simulink model "ROS2ValetPathPlannerExample"  (R2022b)
settings: Solver=FixedStepAuto  StartTime=0.0  StopTime=inf  RelTol=1e-3
model workspace (MAT data in the model file):
  SL_ROS_VariableLengthArrays_MaxSizes.CommonInfo.ArrayTruncateAction = 'EmitWarning'
  SL_ROS_VariableLengthArrays_MaxSizes.MsgTypeMap = containers.Map
  SL_ROS_VariableLengthArrays_MaxSizes.MsgTypeMap.serialization.keys = {'std_msgs/Float64MultiArray'}
  SL_ROS_VariableLengthArrays_MaxSizes.MsgTypeMap.serialization.values{1}.PropertyName = 'data'
  SL_ROS_VariableLengthArrays_MaxSizes.MsgTypeMap.serialization.values{1}.DataType = 'double'
  SL_ROS_VariableLengthArrays_MaxSizes.MsgTypeMap.serialization.values{1}.MaxLength = 1500
  SL_ROS_VariableLengthArrays_MaxSizes.MsgTypeMap.serialization.uniformity = 0
  SL_ROS_VariableLengthArrays_MaxSizes.MsgTypeMap.serialization.keyType = 'char'
  SL_ROS_VariableLengthArrays_MaxSizes.MsgTypeMap.serialization.valueType = 'any'
values from neighbouring files (symbols this model uses):
  costmap = vehicleCostmap(combinedMap, 'CellSize', res)    [exampleHelperROSValetSLCreateCostmap.m]    (also in exampleHelperROSValetSLVisualizePath.m = vehicleCostmap(costmapStruct.Costs,          'FreeThreshold')
  costmapStruct = rmfield(costmapStruct, 'CollisionChecker')    [exampleHelperROSValetSLCreateUtilityStruct.m]
  directions = obj.DirectionsInternal    [ExampleHelperROSValetPathAnalyzer.m]
  vehicleDimsStruct = exampleHelperROSValetMatchStructFields(vehicleDimsStruct, obj.CollisionChecker.VehicleDimensions)    [exampleHelperROSValetSLCreateUtilityStruct.m]
undefined symbols (not defined in the file or in its folder): data, data_SL_Info
libraries: ros2lib x13, drivinglib x2, helperVarsizeLib x1, simulink x1
settings Model: Creator=The MathWorks, Inc.  LastModifiedBy=The MathWorks, Inc.
settings SolverCC: AlgebraicLoopSolver=TrustRegion
settings OptimizationCC: EnhancedBackFolding=on  PassReuseOutputArgsAs=Individual arguments  ZeroExternalMemoryAtStartup=off  ZeroInternalMemoryAtStartup=off  MaxStackSize=64  OptimizeBlockOrder=speed  DifferentSizesBufferReuse=on  OptimizationCustomize=off  EfficientTunableParamExpr=on
settings DebuggingCC: ParameterTunabilityLossMsg=error  UnconnectedInputMsg=warning  UnconnectedOutputMsg=warning  UnconnectedLineMsg=warning  SFMachineParentedDataDiag=warning
settings ModelReferenceCC: EnableRefExpFcnMdlSchedulingChecks=on
settings SFSimCC: SimTargetLang=C++
settings RTWCC: Description=Embedded Coder  SystemTargetFile=ert.tlc  HardwareBoard=Robot Operating System 2 (ROS 2)  TLCOptions=-aInlineSetEventsForThisBaseRateFcn=TLC_FALSE -aSuppressMultiTaskScheduler=TLC_FALSE -aRateBasedStepFcn=1  TemplateMakefile=ert_default_tmf  GenerateReport=on  Toolchain=Colcon Tools  IncludeHyperlinkInReport=on  LaunchReport=on  TargetLang=C++  GenerateTraceInfo=on  GenerateTraceReport=on  GenerateTraceReportSl=on  GenerateTraceReportSf=on  GenerateTraceReportEml=on
settings CodeAppCC: ForceParamTrailComments=on  IgnoreCustomStorageClasses=off  OperatorAnnotations=on  SimulinkDataObjDesc=on  SFDataObjDesc=on  InsertBlockDesc=on
settings ERTTargetCC: SupportVariableSizeSignals=on  RootIOFormat=Structure reference

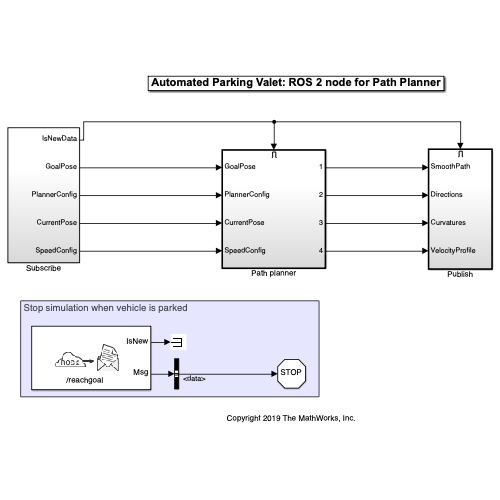
[thumbnail: Simulink's stored preview of the top-level diagram]
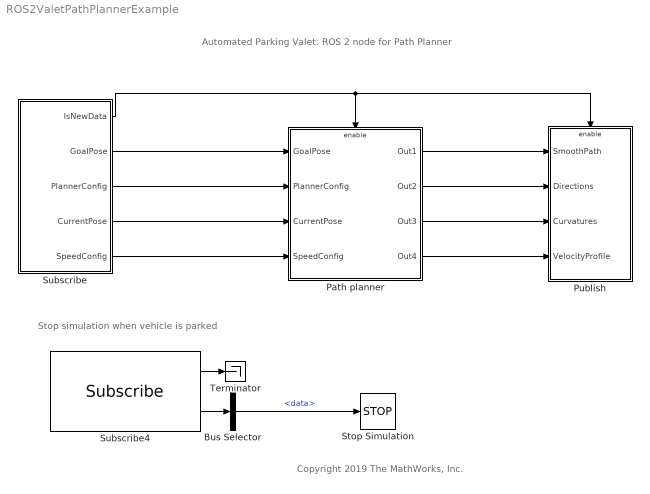
== system ROS2ValetPathPlannerExample ==
  note: Copyright 2019 The MathWorks, Inc.
  note: Automated Parking Valet: ROS 2 node for Path Planner
  note: Stop simulation when vehicle is parked
  Bus Selector : BusSelector  OutputSignals=data
  Path planner : Subsystem
  Publish : Subsystem
  Stop Simulation : Stop
  Subscribe : Subsystem
  Subscribe4 : ros2lib/Subscribe  topicSource=Specify your own  topic=/reachgoal  messageType=std_msgs/Bool  sampleTime=-1  QOSHistory=Keep last  QOSDepth=1  QOSReliability=Reliable  QOSDurability=Volatile
  Terminator : Terminator
  wires:
  Subscribe/2(GoalPose) -> Path planner/1(GoalPose)
  Subscribe/3(PlannerConfig) -> Path planner/2(PlannerConfig)
  Subscribe/1(IsNewData) -> Publish/Enable, Path planner/Enable
  Subscribe/5(SpeedConfig) -> Path planner/4(SpeedConfig)
  Subscribe/4(CurrentPose) -> Path planner/3(CurrentPose)
  Path planner/1(Out1) -> Publish/1(SmoothPath)
  Path planner/2(Out2) -> Publish/2(Directions)
  Path planner/3(Out3) -> Publish/3(Curvatures)
  Path planner/4(Out4) -> Publish/4(VelocityProfile)
  Subscribe4/1 -> Terminator/1
  Bus Selector/1 -> Stop Simulation/1  "<data>"
  Subscribe4/2 -> Bus Selector/1

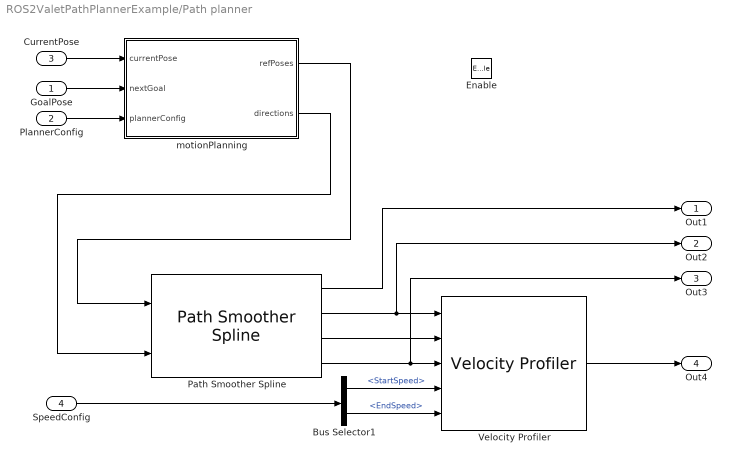
== system ROS2ValetPathPlannerExample/Path planner ==
  GoalPose : Inport
  PlannerConfig : Inport  Port=2
  CurrentPose : Inport  Port=3
  SpeedConfig : Inport  Port=4
  Enable : EnablePort  PropagateVarSize=During execution
  Bus Selector1 : BusSelector  OutputSignals=StartSpeed,EndSpeed
  Path Smoother Spline : drivinglib/Path Smoother Spline  NumSmoothPoses=500  MinSeparation=1e-3  SampleTime=-1  ShowOptionalOutports=on  SimulateUsing=Interpreted execution
  Velocity Profiler : drivinglib/Velocity Profiler  MaxLongitudinalAccel=3  MaxLongitudinalDecel=6  MaxSpeed=10  MaxLongitudinalJerk=1  MaxLateralAccel=3  ShowOptionalOutport=off  SampleTime=-1  SimulateUsing=Interpreted execution
  motionPlanning : MATLAB Function  TreatAsAtomicUnit=on  mask{Costmap=costmap}
      mask prompts: Costmap "Vehicle costmap:"
      mask init:
      | validateattributes(Costmap, {'vehicleCostmap'}, {'scalar'});
      | 
      | [vehicleDimsStruct, costmapStruct] = exampleHelperROSValetSLCreateUtilityStruct(Costmap);
  Out1 : Outport
  Out2 : Outport  Port=2
  Out3 : Outport  Port=3
  Out4 : Outport  Port=4
  wires:
  motionPlanning/1(refPoses) -> Path Smoother Spline/1
  SpeedConfig/1 -> Bus Selector1/1
  Bus Selector1/1 -> Velocity Profiler/4  "<StartSpeed>"
  motionPlanning/2(directions) -> Path Smoother Spline/2
  Bus Selector1/2 -> Velocity Profiler/5  "<EndSpeed>"
  GoalPose/1 -> motionPlanning/2(nextGoal)
  PlannerConfig/1 -> motionPlanning/3(plannerConfig)
  Velocity Profiler/1 -> Out4/1
  CurrentPose/1 -> motionPlanning/1(currentPose)
  Path Smoother Spline/2 -> Out2/1, Velocity Profiler/1
  Path Smoother Spline/3 -> Velocity Profiler/2
  Path Smoother Spline/4 -> Out3/1, Velocity Profiler/3
  Path Smoother Spline/1 -> Out1/1

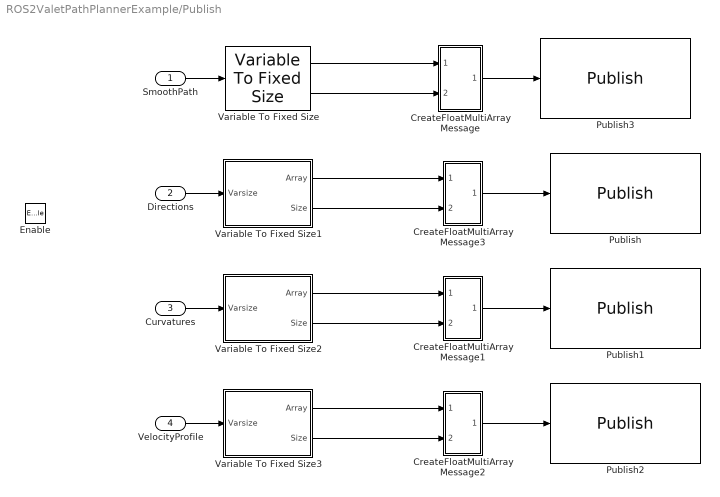
== system ROS2ValetPathPlannerExample/Publish ==
  SmoothPath : Inport
  Directions : Inport  Port=2
  Curvatures : Inport  Port=3
  VelocityProfile : Inport  Port=4
  Enable : EnablePort
  CreateFloatMultiArrayMessage : Subsystem
  CreateFloatMultiArrayMessage1 : Subsystem
  CreateFloatMultiArrayMessage2 : Subsystem
  CreateFloatMultiArrayMessage3 : Subsystem
  Publish : ros2lib/Publish  topicSource=Specify your own  topic=/directions  messageType=std_msgs/Float64MultiArray  QOSHistory=Keep last  QOSDepth=1  QOSReliability=Reliable  QOSDurability=Volatile
  Publish1 : ros2lib/Publish  topicSource=Specify your own  topic=/curvatures  messageType=std_msgs/Float64MultiArray  QOSHistory=Keep last  QOSDepth=1  QOSReliability=Reliable  QOSDurability=Volatile
  Publish2 : ros2lib/Publish  topicSource=Specify your own  topic=/velprofile  messageType=std_msgs/Float64MultiArray  QOSHistory=Keep last  QOSDepth=1  QOSReliability=Reliable  QOSDurability=Volatile
  Publish3 : ros2lib/Publish  topicSource=Specify your own  topic=/smoothpath  messageType=std_msgs/Float64MultiArray  QOSHistory=Keep last  QOSDepth=1  QOSReliability=Reliable  QOSDurability=Volatile
  Variable To Fixed Size : helperVarsizeLib/Variable To Fixed Size  SystemSampleTime=-1  VariantActivationTime=update diagram  Latency=0  AutoFrameSizeCalculation=off
  Variable To Fixed Size1 : Subsystem
  Variable To Fixed Size2 : Subsystem
  Variable To Fixed Size3 : Subsystem
  wires:
  Variable To Fixed Size/1 -> CreateFloatMultiArrayMessage/1(In1)
  Variable To Fixed Size2/2(Size) -> CreateFloatMultiArrayMessage1/2(In2)
  CreateFloatMultiArrayMessage/1(Out1) -> Publish3/1
  Variable To Fixed Size1/1(Array) -> CreateFloatMultiArrayMessage3/1(In1)
  Variable To Fixed Size2/1(Array) -> CreateFloatMultiArrayMessage1/1(In1)
  Variable To Fixed Size1/2(Size) -> CreateFloatMultiArrayMessage3/2(In2)
  CreateFloatMultiArrayMessage2/1(Out1) -> Publish2/1
  CreateFloatMultiArrayMessage1/1(Out1) -> Publish1/1
  CreateFloatMultiArrayMessage3/1(Out1) -> Publish/1
  Variable To Fixed Size/2 -> CreateFloatMultiArrayMessage/2(In2)
  VelocityProfile/1 -> Variable To Fixed Size3/1(Varsize)
  Variable To Fixed Size3/1(Array) -> CreateFloatMultiArrayMessage2/1(In2)
  Variable To Fixed Size3/2(Size) -> CreateFloatMultiArrayMessage2/2(In3)
  Directions/1 -> Variable To Fixed Size1/1(Varsize)
  Curvatures/1 -> Variable To Fixed Size2/1(Varsize)
  SmoothPath/1 -> Variable To Fixed Size/1

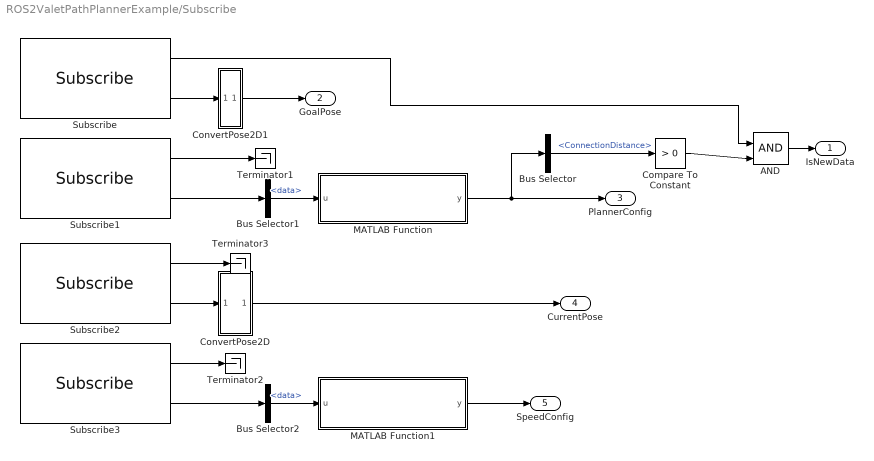
== system ROS2ValetPathPlannerExample/Subscribe ==
  AND : Logic  IconShape=distinctive  AllPortsSameDT=off  OutDataTypeStr=boolean
  Bus Selector : BusSelector  OutputSignals=ConnectionDistance
  Bus Selector1 : BusSelector  OutputSignals=data
  Bus Selector2 : BusSelector  OutputSignals=data
  Compare To Constant : simulink/Logic and Bit Operations/Compare To Constant  relop=>  const=0  OutDataTypeStr=boolean
  ConvertPose2D : Subsystem
  ConvertPose2D1 : Subsystem
  MATLAB Function : MATLAB Function  TreatAsAtomicUnit=on
  MATLAB Function1 : MATLAB Function  TreatAsAtomicUnit=on
  Subscribe : ros2lib/Subscribe  topicSource=Specify your own  topic=/nextgoal  messageType=geometry_msgs/Pose2D  sampleTime=-1  QOSHistory=Keep last  QOSDepth=1  QOSReliability=Reliable  QOSDurability=Volatile
  Subscribe1 : ros2lib/Subscribe  topicSource=Specify your own  topic=/plannerConfig  messageType=std_msgs/Float64MultiArray  sampleTime=-1  QOSHistory=Keep last  QOSDepth=1  QOSReliability=Reliable  QOSDurability=Volatile
  Subscribe2 : ros2lib/Subscribe  topicSource=Specify your own  topic=/currentpose  messageType=geometry_msgs/Pose2D  sampleTime=-1  QOSHistory=Keep last  QOSDepth=1  QOSReliability=Reliable  QOSDurability=Volatile
  Subscribe3 : ros2lib/Subscribe  topicSource=Specify your own  topic=/speed  messageType=std_msgs/Float64MultiArray  sampleTime=-1  QOSHistory=Keep last  QOSDepth=1  QOSReliability=Reliable  QOSDurability=Volatile
  Terminator1 : Terminator
  Terminator2 : Terminator
  Terminator3 : Terminator
  IsNewData : Outport
  GoalPose : Outport  Port=2
  PlannerConfig : Outport  Port=3
  CurrentPose : Outport  Port=4
  SpeedConfig : Outport  Port=5
  wires:
  Subscribe1/1 -> Terminator1/1
  Subscribe2/1 -> Terminator3/1
  Subscribe3/1 -> Terminator2/1
  Subscribe/1 -> AND/1
  Subscribe/2 -> ConvertPose2D1/1(In1)
  Subscribe1/2 -> Bus Selector1/1
  Subscribe3/2 -> Bus Selector2/1
  Subscribe2/2 -> ConvertPose2D/1(In1)
  ConvertPose2D/1(Out1) -> CurrentPose/1
  ConvertPose2D1/1(Out1) -> GoalPose/1
  Bus Selector1/1 -> MATLAB Function/1(u)  "<data>"
  Bus Selector2/1 -> MATLAB Function1/1(u)  "<data>"
  MATLAB Function1/1(y) -> SpeedConfig/1
  MATLAB Function/1(y) -> PlannerConfig/1, Bus Selector/1
  Bus Selector/1 -> Compare To Constant/1  "<ConnectionDistance>"
  Compare To Constant/1 -> AND/2
  AND/1 -> IsNewData/1

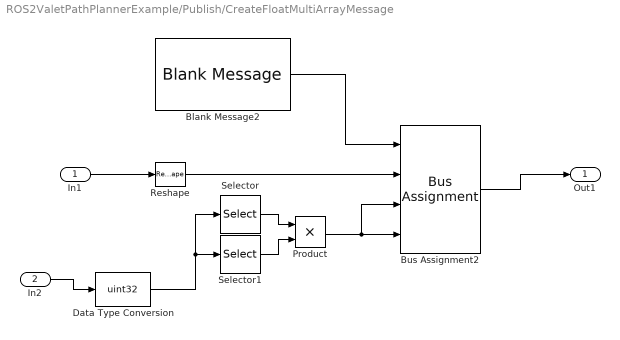
== system ROS2ValetPathPlannerExample/Publish/CreateFloatMultiArrayMessage ==
  In1 : Inport
  In2 : Inport  Port=2
  Blank Message2 : ros2lib/Blank Message  messageClass=Message  entityType=std_msgs/Float64MultiArray  messageType=std_msgs/Float64MultiArray  SampleTime=-1
  Bus Assignment2 : BusAssignment  AssignedSignals=data,data_SL_Info.CurrentLength,data_SL_Info.ReceivedLength
  Data Type Conversion : DataTypeConversion  OutDataTypeStr=uint32  SaturateOnIntegerOverflow=off  RndMeth=Floor
  Product : Product  OutDataTypeStr=uint32
  Reshape : Reshape
  Selector : Selector  InputPortWidth=2  IndexOptions=Index vector (dialog)  Indices=1  OutputSizes=1
  Selector1 : Selector  InputPortWidth=2  IndexOptions=Index vector (dialog)  Indices=2  OutputSizes=1
  Out1 : Outport
  wires:
  In2/1 -> Data Type Conversion/1
  Blank Message2/1 -> Bus Assignment2/1
  Bus Assignment2/1 -> Out1/1
  In1/1 -> Reshape/1
  Reshape/1 -> Bus Assignment2/2
  Selector/1 -> Product/1
  Data Type Conversion/1 -> Selector1/1, Selector/1
  Product/1 -> Bus Assignment2/3, Bus Assignment2/4
  Selector1/1 -> Product/2

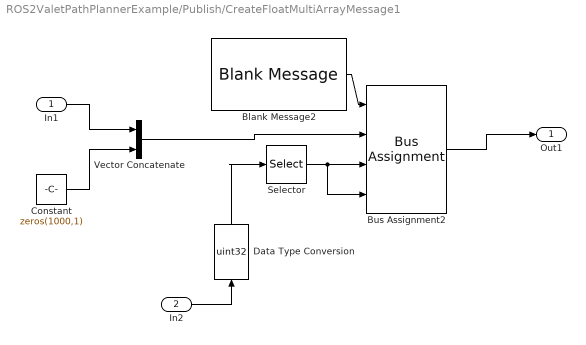
== system ROS2ValetPathPlannerExample/Publish/CreateFloatMultiArrayMessage1 ==
  In1 : Inport
  In2 : Inport  Port=2
  Blank Message2 : ros2lib/Blank Message  messageClass=Message  entityType=std_msgs/Float64MultiArray  messageType=std_msgs/Float64MultiArray  SampleTime=-1
  Bus Assignment2 : BusAssignment  AssignedSignals=data,data_SL_Info.CurrentLength,data_SL_Info.ReceivedLength
  Constant : Constant  Value=zeros(1000,1)
  Data Type Conversion : DataTypeConversion  OutDataTypeStr=uint32  SaturateOnIntegerOverflow=off  RndMeth=Floor
  Selector : Selector  InputPortWidth=2  IndexOptions=Index vector (dialog)  Indices=1  OutputSizes=1
  Vector Concatenate : Concatenate
  Out1 : Outport
  wires:
  Bus Assignment2/1 -> Out1/1
  In1/1 -> Vector Concatenate/1
  Blank Message2/1 -> Bus Assignment2/1
  In2/1 -> Data Type Conversion/1
  Selector/1 -> Bus Assignment2/3, Bus Assignment2/4
  Constant/1 -> Vector Concatenate/2
  Vector Concatenate/1 -> Bus Assignment2/2
  Data Type Conversion/1 -> Selector/1

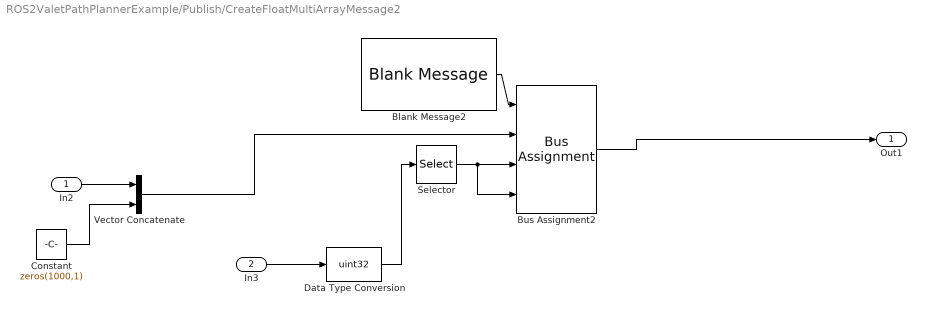
== system ROS2ValetPathPlannerExample/Publish/CreateFloatMultiArrayMessage2 ==
  In2 : Inport
  In3 : Inport  Port=2
  Blank Message2 : ros2lib/Blank Message  messageClass=Message  entityType=std_msgs/Float64MultiArray  messageType=std_msgs/Float64MultiArray  SampleTime=-1
  Bus Assignment2 : BusAssignment  AssignedSignals=data,data_SL_Info.CurrentLength,data_SL_Info.ReceivedLength
  Constant : Constant  Value=zeros(1000,1)
  Data Type Conversion : DataTypeConversion  OutDataTypeStr=uint32  SaturateOnIntegerOverflow=off  RndMeth=Floor
  Selector : Selector  InputPortWidth=2  IndexOptions=Index vector (dialog)  Indices=1  OutputSizes=1
  Vector Concatenate : Concatenate
  Out1 : Outport
  wires:
  Blank Message2/1 -> Bus Assignment2/1
  Bus Assignment2/1 -> Out1/1
  Vector Concatenate/1 -> Bus Assignment2/2
  Constant/1 -> Vector Concatenate/2
  Selector/1 -> Bus Assignment2/4, Bus Assignment2/3
  In3/1 -> Data Type Conversion/1
  In2/1 -> Vector Concatenate/1
  Data Type Conversion/1 -> Selector/1

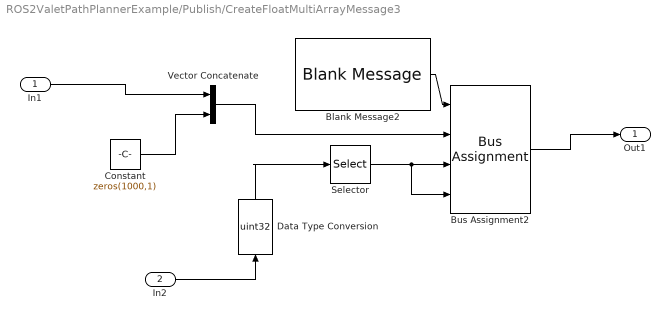
== system ROS2ValetPathPlannerExample/Publish/CreateFloatMultiArrayMessage3 ==
  In1 : Inport
  In2 : Inport  Port=2
  Blank Message2 : ros2lib/Blank Message  messageClass=Message  entityType=std_msgs/Float64MultiArray  messageType=std_msgs/Float64MultiArray  SampleTime=-1
  Bus Assignment2 : BusAssignment  AssignedSignals=data,data_SL_Info.CurrentLength,data_SL_Info.ReceivedLength
  Constant : Constant  Value=zeros(1000,1)
  Data Type Conversion : DataTypeConversion  OutDataTypeStr=uint32  SaturateOnIntegerOverflow=off  RndMeth=Floor
  Selector : Selector  InputPortWidth=2  IndexOptions=Index vector (dialog)  Indices=1  OutputSizes=1
  Vector Concatenate : Concatenate
  Out1 : Outport
  wires:
  Bus Assignment2/1 -> Out1/1
  Blank Message2/1 -> Bus Assignment2/1
  In2/1 -> Data Type Conversion/1
  Selector/1 -> Bus Assignment2/3, Bus Assignment2/4
  Constant/1 -> Vector Concatenate/2
  In1/1 -> Vector Concatenate/1
  Vector Concatenate/1 -> Bus Assignment2/2
  Data Type Conversion/1 -> Selector/1

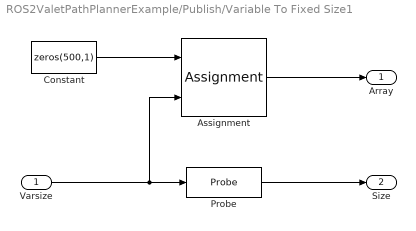
== system ROS2ValetPathPlannerExample/Publish/Variable To Fixed Size1 ==
  Varsize : Inport
  Assignment : Assignment  NumberOfDimensions=2  IndexMode=Zero-based  DiagnosticForDimensions=Warning  IndexOptions=Starting index (dialog),Starting index (dialog)  Indices=0,0  OutputSizes=1,1
  Constant : Constant  Value=zeros(500,1)  VectorParams1D=off
  Probe : Probe  ProbeWidth=off  ProbeSampleTime=off  ProbeComplexSignal=off  ProbeSignalDimensions=on
  Array : Outport  VectorParamsAs1DForOutWhenUnconnected=off
  Size : Outport  Port=2  VectorParamsAs1DForOutWhenUnconnected=off
  wires:
  Constant/1 -> Assignment/1
  Varsize/1 -> Probe/1, Assignment/2
  Assignment/1 -> Array/1
  Probe/1 -> Size/1

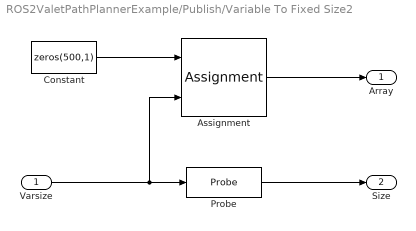
== system ROS2ValetPathPlannerExample/Publish/Variable To Fixed Size2 ==
  Varsize : Inport
  Assignment : Assignment  NumberOfDimensions=2  IndexMode=Zero-based  DiagnosticForDimensions=Warning  IndexOptions=Starting index (dialog),Starting index (dialog)  Indices=0,0  OutputSizes=1,1
  Constant : Constant  Value=zeros(500,1)  VectorParams1D=off
  Probe : Probe  ProbeWidth=off  ProbeSampleTime=off  ProbeComplexSignal=off  ProbeSignalDimensions=on
  Array : Outport  VectorParamsAs1DForOutWhenUnconnected=off
  Size : Outport  Port=2  VectorParamsAs1DForOutWhenUnconnected=off
  wires:
  Constant/1 -> Assignment/1
  Varsize/1 -> Probe/1, Assignment/2
  Assignment/1 -> Array/1
  Probe/1 -> Size/1

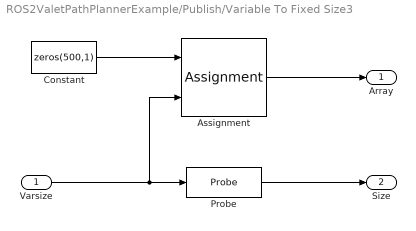
== system ROS2ValetPathPlannerExample/Publish/Variable To Fixed Size3 ==
  Varsize : Inport
  Assignment : Assignment  NumberOfDimensions=2  IndexMode=Zero-based  DiagnosticForDimensions=Warning  IndexOptions=Starting index (dialog),Starting index (dialog)  Indices=0,0  OutputSizes=1,1
  Constant : Constant  Value=zeros(500,1)  VectorParams1D=off
  Probe : Probe  ProbeWidth=off  ProbeSampleTime=off  ProbeComplexSignal=off  ProbeSignalDimensions=on
  Array : Outport  VectorParamsAs1DForOutWhenUnconnected=off
  Size : Outport  Port=2  VectorParamsAs1DForOutWhenUnconnected=off
  wires:
  Probe/1 -> Size/1
  Assignment/1 -> Array/1
  Varsize/1 -> Assignment/2, Probe/1
  Constant/1 -> Assignment/1

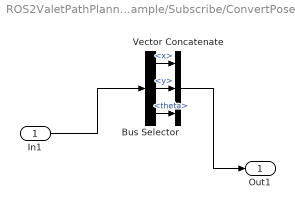
== system ROS2ValetPathPlannerExample/Subscribe/ConvertPose2D ==
  In1 : Inport
  Bus Selector : BusSelector  OutputSignals=x,y,theta
  Vector Concatenate : Concatenate  NumInputs=3
  Out1 : Outport
  wires:
  Vector Concatenate/1 -> Out1/1
  Bus Selector/1 -> Vector Concatenate/1  "<x>"
  In1/1 -> Bus Selector/1
  Bus Selector/3 -> Vector Concatenate/3  "<theta>"
  Bus Selector/2 -> Vector Concatenate/2  "<y>"

== system ROS2ValetPathPlannerExample/Subscribe/ConvertPose2D1 ==
  In1 : Inport
  Bus Selector : BusSelector  OutputSignals=x,y,theta
  Vector Concatenate : Concatenate  NumInputs=3
  Out1 : Outport
  wires:
  Vector Concatenate/1 -> Out1/1
  Bus Selector/1 -> Vector Concatenate/1  "<x>"
  In1/1 -> Bus Selector/1
  Bus Selector/3 -> Vector Concatenate/3  "<theta>"
  Bus Selector/2 -> Vector Concatenate/2  "<y>"

== matlab function ROS2ValetPathPlannerExample/Path planner/motionPlanning ==
  settings: updateMethod=DISCRETE  sampleTime=0.1
  data: refPoses output size=[100 3]; currentPose input size=[1 3]; nextGoal input size=[1 3]; plannerConfig input Bus: plannerConfigBus; costmapStruct parameter; vehicleDimsStruct parameter; directions output size=[100 1]
function [refPoses, directions] = motionPlanning(currentPose, nextGoal, ...
    plannerConfig, costmapStruct, vehicleDimsStruct)

%motionPlanning plan a feasible path using pathPlannerRRT.

%#codegen

persistent nextGoalPose posesInternal directionsInternal 

% Initialize persistent variables
if isempty(nextGoalPose)
    nextGoalPose = [0 0 0];
end

if isempty(posesInternal)
    posesInternal = [0 0 0];
end

if isempty(directionsInternal)
    directionsInternal = 1;
end

% Create vehicleDimensions object
vehicleDims = vehicleDimensions( ...
    vehicleDimsStruct.Length, ...
    vehicleDimsStruct.Width, ...
    vehicleDimsStruct.Height, ...
    'Wheelbase',          vehicleDimsStruct.Wheelbase, ...
    'RearOverhang',       vehicleDimsStruct.RearOverhang, ...
    'WorldUnits',         char(vehicleDimsStruct.WorldUnits));

ccConfig = inflationCollisionChecker(vehicleDims, 4);

% Initialize vehicleCostmap object
costmap = vehicleCostmap(costmapStruct.Costs, ...
    'FreeThreshold',      costmapStruct.FreeThreshold, ...
    'OccupiedThreshold',  costmapStruct.OccupiedThreshold, ...
    'MapLocation',        costmapStruct.MapExtent([1, 3]), ...
    'CellSize',           costmapStruct.CellSize, ...
    'CollisionChecker',   ccConfig);

% Create pathPlannerRRT object
motionPlanner = pathPlannerRRT(costmap, ...
    'ConnectionDistance', plannerConfig.ConnectionDistance, ...
    'MinIterations',      plannerConfig.MinIterations, ...
    'GoalTolerance',      plannerConfig.GoalTolerance, ...
    'MinTurningRadius',   plannerConfig.MinTurningRadius);

% Only plan the path if there is a new goal
if ~isequal(nextGoalPose, nextGoal)
    nextGoalPose  = nextGoal;
    vehiclePose   = currentPose;
    refPath       = plan(motionPlanner, vehiclePose, nextGoalPose);
    pathLength    = refPath.Length;
    while((pathLength  == 0) || (pathLength > 80))
        refPath       = plan(motionPlanner, vehiclePose, nextGoalPose);
        pathLength    = refPath.Length;
    end
    [refPoses, directions] = interpolate(refPath);
    posesInternal          = refPoses;
    directionsInternal     = directions;
else
    refPoses   = posesInternal;
    directions = directionsInternal;
end

end

== matlab function ROS2ValetPathPlannerExample/Subscribe/MATLAB Function ==
  data: y output Bus: plannerConfigBus; u input
function y = extractPlannerConfigBus(u)
y.ConnectionDistance =  u(1);
y.MinIterations = u(2);
y.GoalTolerance  = u(3:5)';
y.MinTurningRadius = u(6);

== matlab function ROS2ValetPathPlannerExample/Subscribe/MATLAB Function1 ==
  data: y output Bus: speedConfigBus; u input
function y = extractSpeedConfigBus(u)
y.StartSpeed =  u(1);
y.EndSpeed = u(2);
y.MaxSpeed  = u(3);
